simulink model "ejercicio3"  (R2021b)
settings: Solver=VariableStepAuto  StartTime=0.0  StopTime=10.0  MaxStep=0.1  RelTol=1e-3
libraries: fuzblock x1
settings Model: Creator=Daniel  LastModifiedBy=Daniel

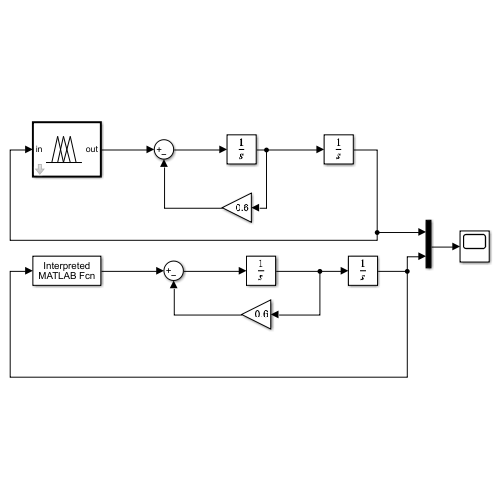
[thumbnail: Simulink's stored preview of the top-level diagram]
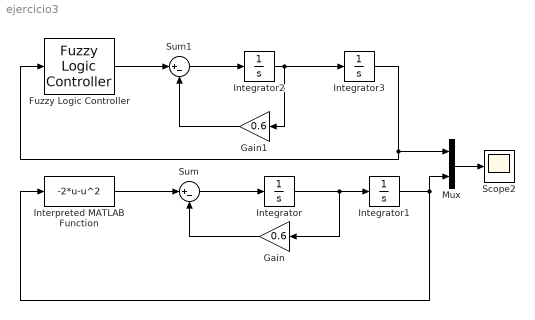
== system ejercicio3 ==
  Fuzzy Logic Controller : fuzblock/Fuzzy Logic  Controller  FIS=fismat1  OutputSampleNumber=101  DataType=double  FuzzifiedInputs=off  RuleFiringStrengths=off  RuleOutputs=off  AggregatedOutputs=off  SimulateUsing=Interpreted execution  OutOfRangeInputValueMessage=warning  NoRuleFiredMessage=warning  EmptyOutputFuzzySetMessage=warning
  Gain : Gain  Gain=0.6
  Gain1 : Gain  Gain=0.6
  Integrator : Integrator  InitialCondition=0.5
  Integrator1 : Integrator  InitialCondition=0.2
  Integrator2 : Integrator  InitialCondition=0.5
  Integrator3 : Integrator  InitialCondition=0.2
  Interpreted MATLAB Function : MATLABFcn  MATLABFcn=-2*u-u^2
  Mux : Mux  Inputs=2
  Scope2 : Scope
  Sum : Sum  Inputs=|+-
  Sum1 : Sum  Inputs=|+-
  wires:
  Interpreted MATLAB Function/1 -> Sum/1
  Sum/1 -> Integrator/1
  Integrator/1 -> Gain/1, Integrator1/1
  Gain/1 -> Sum/2
  Integrator1/1 -> Interpreted MATLAB Function/1, Mux/2
  Fuzzy Logic Controller/1 -> Sum1/1
  Sum1/1 -> Integrator2/1
  Integrator2/1 -> Integrator3/1, Gain1/1
  Gain1/1 -> Sum1/2
  Integrator3/1 -> Mux/1, Fuzzy Logic Controller/1
  Mux/1 -> Scope2/1
